simulink model "rpdriver_2018b"  (R2018b)
settings: Solver=FixedStepDiscrete  StartTime=0.0  StopTime=999  FixedStep=0.01  RelTol=1e-3  EnableMultiTasking=on
undefined symbols (not defined in the file or in its folder): K
libraries: powerlib_meascontrol x1
settings Model: SimulationMode=external  ExtModeTrigDuration=30000  Creator=user  LastModifiedBy=Admin
settings DataIOCC: SaveFormat=Array  SignalLoggingSaveFormat=ModelDataLogs
settings OptimizationCC: ExpressionDepthLimit=2147483647  LifeSpan=inf
settings DebuggingCC: UnderspecifiedInitializationDetection=Classic  MergeDetectMultiDrivingBlocksExec=none  SolverPrmCheckMsg=warning  FcnCallInpInsideContextMsg=warning  StateNameClashWarn=warning  SFUnexpectedBacktrackingDiag=warning  SFNoUnconditionalDefaultTransitionDiag=warning  SFExecutionAtInitializationDiag=none
settings HardwareCC: ProdBitPerPointer=32  ProdBitPerSizeT=32  ProdBitPerPtrDiffT=32  ProdLargestAtomicFloat=None  ProdIntDivRoundTo=Undefined  ProdEndianess=Unspecified  ProdWordSize=32  ProdHWDeviceType=32-bit Generic
settings ModelReferenceCC: PropagateSignalLabelsOutOfModel=off
settings SFSimCC: SimUseLocalCustomCode=off
settings RTWCC: Description=rpend RTDAC/USB2 (Visual C/C++)  SystemTargetFile=rtcon_rpend_usb2.tlc  TemplateMakefile=rtcon_rpend_vc_usb2_x64.tmf  RTWUseLocalCustomCode=off
settings CodeAppCC: StateflowObjectComments=on
settings STFCustomTargetCC: ModelReferenceCompliant=off  CombineOutputUpdateFcns=on  MatFileLogging=on  SystemTargetFile=rtcon_rpend_usb2.tlc
settings GRTTargetCC: TargetLangStandard=C89/C90 (ANSI)  ModelReferenceCompliant=off  ParMdlRefBuildCompliant=off  CompOptLevelCompliant=off  ConcurrentExecutionCompliant=off  CPPClassGenCompliant=off  UseToolchainInfoCompliant=off  ExtMode=on  ExtModeMexFile=rtcon_ext_comm
settings ConfigComp: CovMetricSettings=dw  CovSaveCumulativeToWorkspaceVar=on  CovSaveSingleToWorkspaceVar=on  CovExternalEMLEnable=off  CovSFcnEnable=off

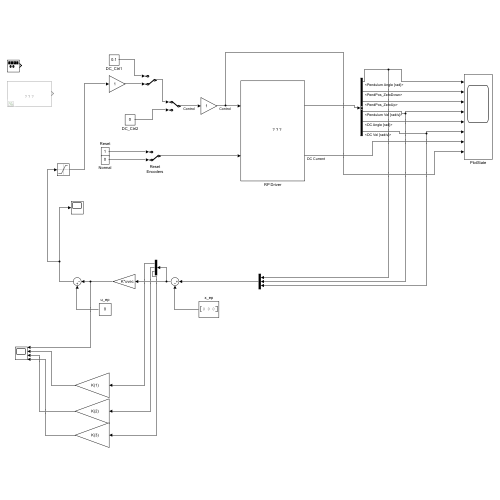
[thumbnail: Simulink's stored preview of the top-level diagram]
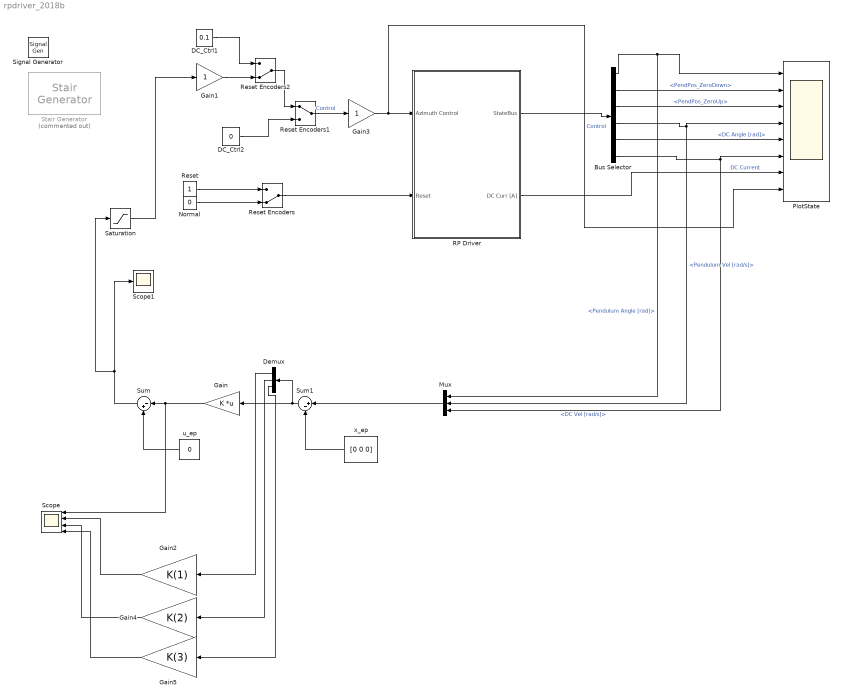
== system rpdriver_2018b ==
  Bus Selector : BusSelector  OutputSignals=Pendulum Angle [rad],PendPos_ZeroDown,PendPos_ZeroUp,Pendulum Vel [rad/s],DC Angle [rad],DC Vel [rad/s]
  DC_Ctrl1 : Constant  Value=0.1
  DC_Ctrl2 : Constant  Value=0
  Demux : Demux  Outputs=3
  Gain : Gain  Gain=K  Multiplication=Matrix(K*u) (u vector)
  Gain1 : Gain
  Gain2 : Gain  Gain=K(1)
  Gain3 : Gain
  Gain4 : Gain  Gain=K(2)
  Gain5 : Gain  Gain=K(3)
  Mux : Mux  Inputs=3
  Normal : Constant  Value=0
  PlotState : Scope  NumInputPorts=8
  RP Driver : Subsystem
      mask Display: image(imread('rwp.JPG'))
  Reset : Constant
  Reset Encoders : ManualSwitch  CurrentSetting=0
  Reset Encoders1 : ManualSwitch
  Reset Encoders2 : ManualSwitch  CurrentSetting=0
  Saturation : Saturate  UpperLimit=0.9  LowerLimit=-0.9
  Scope : Scope  NumInputPorts=4
  Scope1 : Scope
  Signal Generator : SignalGenerator  WaveForm=square  Amplitude=0.25  Frequency=1/9
  Stair Generator : powerlib_meascontrol/Pulse & Signal Generators/Stair Generator  Commented=on  t=time  e=amp  Ts=0
  Sum : Sum  Inputs=|-+
  Sum1 : Sum  Inputs=|+-
  u_ep : Constant  Value=0
  x_ep : Constant  Value=[0 0 0]
  wires:
  Normal/1 -> Reset Encoders/2
  Reset/1 -> Reset Encoders/1
  Reset Encoders/1 -> RP Driver/2(Reset)
  RP Driver/1(StateBus) -> Bus Selector/1
  Reset Encoders1/1 -> Gain3/1  "Control"
  DC_Ctrl1/1 -> Reset Encoders2/1
  Reset Encoders2/1 -> Reset Encoders1/1
  Gain1/1 -> Reset Encoders2/2
  Gain3/1 -> PlotState/8, RP Driver/1(Azimuth Control)  "Control"
  DC_Ctrl2/1 -> Reset Encoders1/2
  Bus Selector/1 -> Mux/1, PlotState/1  "<Pendulum Angle [rad]>"
  Bus Selector/2 -> PlotState/2  "<PendPos_ZeroDown>"
  Bus Selector/3 -> PlotState/3  "<PendPos_ZeroUp>"
  Bus Selector/4 -> Mux/2, PlotState/4  "<Pendulum Vel [rad/s]>"
  Bus Selector/5 -> PlotState/5  "<DC Angle [rad]>"
  Bus Selector/6 -> Mux/3, PlotState/6  "<DC Vel [rad/s]>"
  RP Driver/2(DC Curr [A]) -> PlotState/7  "DC Current"
  x_ep/1 -> Sum1/2
  u_ep/1 -> Sum/2
  Sum/1 -> Saturation/1, Scope1/1
  Mux/1 -> Sum1/1
  Gain/1 -> Scope/1, Sum/1
  Sum1/1 -> Demux/1, Gain/1
  Demux/1 -> Gain2/1
  Demux/2 -> Gain4/1
  Demux/3 -> Gain5/1
  Gain2/1 -> Scope/2
  Gain4/1 -> Scope/3
  Gain5/1 -> Scope/4
  Saturation/1 -> Gain1/1

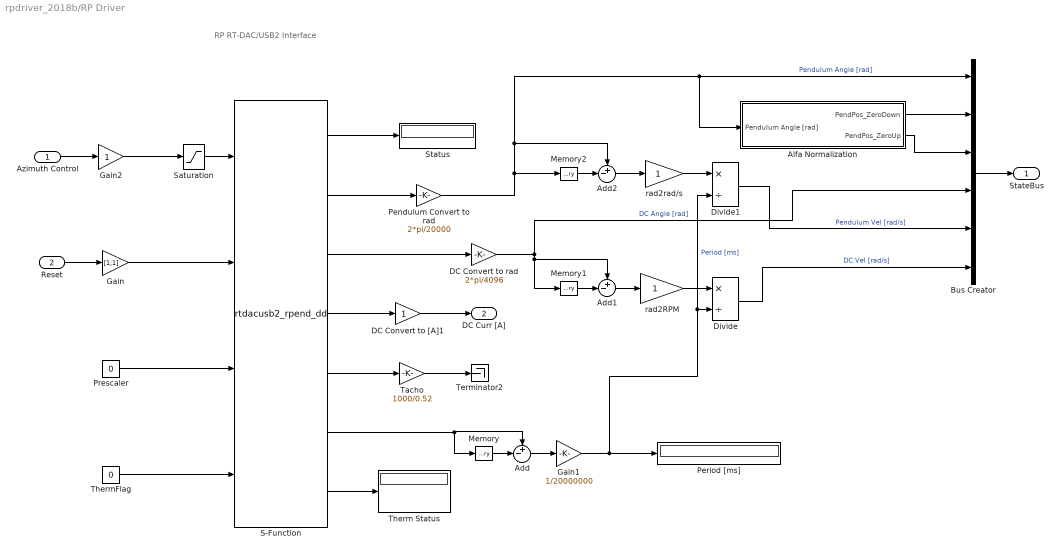
== system rpdriver_2018b/RP Driver ==
  note: RP RT-DAC/USB2
      | Interface
  Azimuth Control : Inport
  Reset : Inport  Port=2
  Add : Sum  Inputs=+-|
  Add1 : Sum  Inputs=+-|
  Add2 : Sum  Inputs=+-|
  Alfa Normalization : Subsystem
  Bus Creator : BusCreator  Inputs=6
  DC Convert to [A]1 : Gain  SaturateOnIntegerOverflow=on  OutDataTypeStr=Inherit: Same as input  ParamDataTypeStr=Inherit: Same as input
  DC Convert to rad : Gain  Gain=2*pi/4096  SaturateOnIntegerOverflow=on  OutDataTypeStr=Inherit: Same as input  ParamDataTypeStr=Inherit: Same as input
  Divide : Product  Inputs=*/
  Divide1 : Product  Inputs=*/
  Gain : Gain  Gain=[1;1]
  Gain1 : Gain  Gain=1/20000000
  Gain2 : Gain
  Memory : Memory
  Memory1 : Memory
  Memory2 : Memory
  Pendulum Convert to rad : Gain  Gain=2*pi/20000  SaturateOnIntegerOverflow=on  OutDataTypeStr=Inherit: Same as input  ParamDataTypeStr=Inherit: Same as input
  Period [ms] : Display
  Prescaler : Constant  Value=0
  S-Function : S-Function  FunctionName=rtdacusb2_rpend_dd  Parameters=1, 0.01  SFunctionDeploymentMode=off  EnableBusSupport=off
  Saturation : Saturate  UpperLimit=1  LowerLimit=-1
  Status : Display
  Tacho : Gain  Gain=1000/0.52  SaturateOnIntegerOverflow=on  OutDataTypeStr=Inherit: Same as input  ParamDataTypeStr=Inherit: Same as input
  Terminator2 : Terminator
  Therm Status : Display
  ThermFlag : Constant  Value=0
  rad2RPM : Gain  SaturateOnIntegerOverflow=on  OutDataTypeStr=Inherit: Same as input  ParamDataTypeStr=Inherit: Same as input
  rad2rad/s : Gain  SaturateOnIntegerOverflow=on  OutDataTypeStr=Inherit: Same as input  ParamDataTypeStr=Inherit: Same as input
  StateBus : Outport  VectorParamsAs1DForOutWhenUnconnected=off
  DC Curr [A] : Outport  Port=2  VectorParamsAs1DForOutWhenUnconnected=off
  wires:
  S-Function/7 -> Therm Status/1
  S-Function/5 -> Tacho/1
  S-Function/4 -> DC Convert to [A]1/1
  ThermFlag/1 -> S-Function/4
  Prescaler/1 -> S-Function/3
  Gain/1 -> S-Function/2
  DC Convert to [A]1/1 -> DC Curr [A]/1
  Divide/1 -> Bus Creator/6  "DC Vel [rad/s]"
  Divide1/1 -> Bus Creator/5  "Pendulum Vel [rad/s]"
  Alfa Normalization/2(PendPos_ZeroUp) -> Bus Creator/3
  Alfa Normalization/1(PendPos_ZeroDown) -> Bus Creator/2
  Bus Creator/1 -> StateBus/1
  rad2rad/s/1 -> Divide1/1
  Add2/1 -> rad2rad/s/1
  Memory2/1 -> Add2/2
  rad2RPM/1 -> Divide/1
  Add1/1 -> rad2RPM/1
  Memory1/1 -> Add1/2
  Tacho/1 -> Terminator2/1
  S-Function/6 -> Add/1, Memory/1
  Gain2/1 -> Saturation/1
  Gain1/1 -> Period [ms]/1, Divide/2, Divide1/2  "Period [ms]"
  Add/1 -> Gain1/1
  Memory/1 -> Add/2
  DC Convert to rad/1 -> Memory1/1, Add1/1, Bus Creator/4  "DC Angle [rad]"
  S-Function/3 -> DC Convert to rad/1
  Pendulum Convert to rad/1 -> Bus Creator/1, Alfa Normalization/1(Pendulum Angle [rad]), Add2/1, Memory2/1  "Pendulum Angle [rad]"
  S-Function/1 -> Status/1
  Saturation/1 -> S-Function/1
  Reset/1 -> Gain/1
  Azimuth Control/1 -> Gain2/1
  S-Function/2 -> Pendulum Convert to rad/1

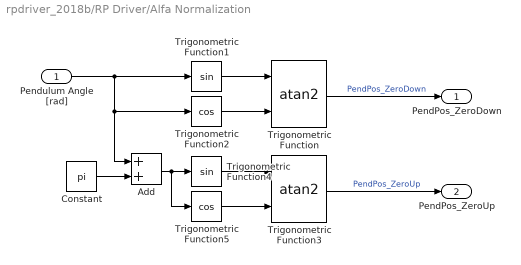
== system rpdriver_2018b/RP Driver/Alfa Normalization ==
  Pendulum Angle [rad] : Inport
  Add : Sum
  Constant : Constant  Value=pi
  Trigonometric Function : Trigonometry  Operator=atan2
  Trigonometric Function1 : Trigonometry
  Trigonometric Function2 : Trigonometry  Operator=cos
  Trigonometric Function3 : Trigonometry  Operator=atan2
  Trigonometric Function4 : Trigonometry
  Trigonometric Function5 : Trigonometry  Operator=cos
  PendPos_ZeroDown : Outport  VectorParamsAs1DForOutWhenUnconnected=off
  PendPos_ZeroUp : Outport  Port=2  VectorParamsAs1DForOutWhenUnconnected=off
  wires:
  Constant/1 -> Add/2
  Add/1 -> Trigonometric Function4/1, Trigonometric Function5/1
  Trigonometric Function5/1 -> Trigonometric Function3/2
  Trigonometric Function4/1 -> Trigonometric Function3/1
  Trigonometric Function3/1 -> PendPos_ZeroUp/1  "PendPos_ZeroUp"
  Trigonometric Function2/1 -> Trigonometric Function/2
  Trigonometric Function1/1 -> Trigonometric Function/1
  Pendulum Angle [rad]/1 -> Add/1, Trigonometric Function2/1, Trigonometric Function1/1
  Trigonometric Function/1 -> PendPos_ZeroDown/1  "PendPos_ZeroDown"
